simulink model "fireSpreading_analysis"  (R2021a)
settings: Solver=VariableStepAuto  StartTime=0.0  StopTime=10.0  RelTol=1e-3
values from neighbouring files (symbols this model uses):
  centroidi2 = cen_input'    [adj_cen.m]
  monitoring_critical_threshold = 15    [variables.m]
  numero_centroidi = col    [adj_cen.m]
  numero_wp = col    [adj_cen.m]
  time_burn_cell = cell_lenght*time_burn_meter    [variables.m]
  time_burn_meter = 20    [variables.m]
undefined symbols (not defined in the file or in its folder): ct, elementi_classe, pt, rt
settings Model: Creator=fiori  LastModifiedBy=fiori
settings SolverCC: AlgebraicLoopSolver=TrustRegion
settings DebuggingCC: SFMachineParentedDataDiag=warning

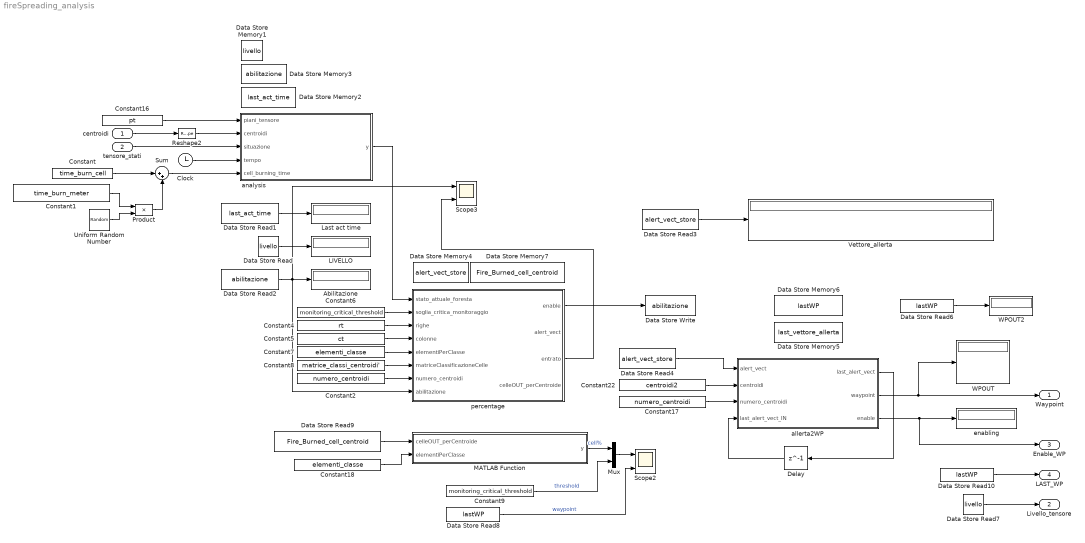
== system fireSpreading_analysis ==
  centroidi : Inport  PortDimensions=[3,numero_centroidi]
  tensore_stati : Inport  Port=2  PortDimensions=[rt,ct,pt]
  Abilitazione : Display
  Clock : Clock
  Constant : Constant  Value=time_burn_cell
  Constant1 : Constant  Value=time_burn_meter
  Constant16 : Constant  Value=pt
  Constant17 : Constant  Value=numero_centroidi
  Constant18 : Constant  Value=elementi_classe
  Constant2 : Constant  Value=numero_centroidi
  Constant22 : Constant  Value=centroidi2
  Constant4 : Constant  Value=rt
  Constant5 : Constant  Value=ct
  Constant6 : Constant  Value=monitoring_critical_threshold
  Constant7 : Constant  Value=elementi_classe
  Constant8 : Constant  Value=matrice_classi_centroidi'
  Constant9 : Constant  Value=monitoring_critical_threshold
  Data Store Memory1 : DataStoreMemory  DataStoreName=livello  ReadBeforeWriteMsg=warning  WriteAfterWriteMsg=warning  WriteAfterReadMsg=warning  ShowAdditionalParam=off  OutDataTypeStr=double
  Data Store Memory2 : DataStoreMemory  DataStoreName=last_act_time  ReadBeforeWriteMsg=warning  WriteAfterWriteMsg=warning  WriteAfterReadMsg=warning  ShowAdditionalParam=off  OutDataTypeStr=double
  Data Store Memory3 : DataStoreMemory  DataStoreName=abilitazione  ReadBeforeWriteMsg=warning  WriteAfterWriteMsg=warning  WriteAfterReadMsg=warning  ShowAdditionalParam=off  OutDataTypeStr=double
  Data Store Memory4 : DataStoreMemory  DataStoreName=alert_vect_store  ReadBeforeWriteMsg=warning  WriteAfterWriteMsg=warning  WriteAfterReadMsg=warning  ShowAdditionalParam=off  OutDataTypeStr=double  Dimensions=[1,numero_centroidi]
  Data Store Memory5 : DataStoreMemory  DataStoreName=last_vettore_allerta  ReadBeforeWriteMsg=warning  WriteAfterWriteMsg=warning  WriteAfterReadMsg=warning  ShowAdditionalParam=off  OutDataTypeStr=double  Dimensions=[1,numero_centroidi]
  Data Store Memory6 : DataStoreMemory  DataStoreName=lastWP  ReadBeforeWriteMsg=warning  WriteAfterWriteMsg=warning  WriteAfterReadMsg=warning  ShowAdditionalParam=off  OutDataTypeStr=double
  Data Store Memory7 : DataStoreMemory  DataStoreName=Fire_Burned_cell_centroid  ReadBeforeWriteMsg=warning  WriteAfterWriteMsg=warning  WriteAfterReadMsg=warning  ShowAdditionalParam=off  OutDataTypeStr=double  Dimensions=[1,numero_centroidi]
  Data Store Read : DataStoreRead  DataStoreName=livello  IndexOptions=Index vector (dialog)  Indices=1  OutputSizes=1
  Data Store Read1 : DataStoreRead  DataStoreName=last_act_time  IndexOptions=Index vector (dialog)  Indices=1  OutputSizes=1
  Data Store Read10 : DataStoreRead  DataStoreName=lastWP  IndexOptions=Index vector (dialog)  Indices=1  OutputSizes=1
  Data Store Read2 : DataStoreRead  DataStoreName=abilitazione  IndexOptions=Index vector (dialog)  Indices=1  OutputSizes=1
  Data Store Read3 : DataStoreRead  DataStoreName=alert_vect_store  IndexOptions=Index vector (dialog)  Indices=1  OutputSizes=1
  Data Store Read4 : DataStoreRead  DataStoreName=alert_vect_store  IndexOptions=Index vector (dialog)  Indices=1  OutputSizes=1
  Data Store Read6 : DataStoreRead  DataStoreName=lastWP  IndexOptions=Index vector (dialog)  Indices=1  OutputSizes=1
  Data Store Read7 : DataStoreRead  DataStoreName=livello  IndexOptions=Index vector (dialog)  Indices=1  OutputSizes=1
  Data Store Read8 : DataStoreRead  DataStoreName=lastWP  IndexOptions=Index vector (dialog)  Indices=1  OutputSizes=1
  Data Store Read9 : DataStoreRead  DataStoreName=Fire_Burned_cell_centroid  IndexOptions=Index vector (dialog)  Indices=1  OutputSizes=1
  Data Store Write : DataStoreWrite  DataStoreName=abilitazione  IndexOptions=Index vector (dialog)  Indices=1  OutputSizes=1
  Delay : Delay  DelayLength=1  InitialCondition=0
  LIVELLO : Display
  Last act time : Display
  MATLAB Function : MATLAB Function  TreatAsAtomicUnit=on
  Mux : Mux  Inputs=2
  Product : Product
  Reshape2 : Reshape  OutputDimensionality=Customize  OutputDimensions=[3,numero_wp]
  Scope2 : Scope  NumInputPorts=2
  Scope3 : Scope  NumInputPorts=3
  Sum : Sum  Inputs=|++
  Uniform Random Number : UniformRandomNumber  SampleTime=0.1
  Vettore_allerta : Display
  WPOUT : Display
  WPOUT2 : Display
  allerta2WP : MATLAB Function  TreatAsAtomicUnit=on
  analysis : MATLAB Function  TreatAsAtomicUnit=on
  enabling : Display
  percentage : MATLAB Function  TreatAsAtomicUnit=on
  Waypoint : Outport
  Livello_tensore : Outport  Port=2
  Enable_WP : Outport  Port=3
  LAST_WP : Outport  Port=4
  wires:
  centroidi/1 -> Reshape2/1
  Clock/1 -> analysis/4(tempo)
  tensore_stati/1 -> analysis/3(situazione)
  Uniform Random Number/1 -> Product/2
  Constant1/1 -> Product/1
  Constant/1 -> Sum/1
  Product/1 -> Sum/2
  analysis/1(y) -> percentage/1(stato_attuale_foresta)
  Reshape2/1 -> analysis/2(centroidi)
  Data Store Read/1 -> LIVELLO/1
  Data Store Read1/1 -> Last act time/1
  Constant6/1 -> percentage/2(soglia_critica_monitoraggio)
  Constant4/1 -> percentage/3(righe)
  Constant5/1 -> percentage/4(colonne)
  Constant7/1 -> percentage/5(elementiPerClasse)
  Constant8/1 -> percentage/6(matriceClassificazioneCelle)
  Constant2/1 -> percentage/7(numero_centroidi)
  Constant22/1 -> allerta2WP/2(centroidi)
  Data Store Read2/1 -> Scope3/1, percentage/8(abilitazione), Abilitazione/1
  percentage/1(enable) -> Data Store Write/1
  percentage/3(entrato) -> Scope3/3
  Data Store Read3/1 -> Vettore_allerta/1
  Constant16/1 -> analysis/1(piani_tensore)
  Data Store Read4/1 -> allerta2WP/1(alert_vect)
  Constant17/1 -> allerta2WP/3(numero_centroidi)
  Delay/1 -> allerta2WP/4(last_alert_vect_IN)
  allerta2WP/1(last_alert_vect) -> Delay/1
  allerta2WP/2(waypoint) -> WPOUT/1, Waypoint/1
  allerta2WP/3(enable) -> enabling/1, Enable_WP/1
  Data Store Read6/1 -> WPOUT2/1
  Data Store Read7/1 -> Livello_tensore/1
  Data Store Read9/1 -> MATLAB Function/1(celleOUT_perCentroide)
  Constant18/1 -> MATLAB Function/2(elementiPerClasse)
  Data Store Read8/1 -> Scope2/2  "waypoint"
  MATLAB Function/1(y) -> Mux/1  "cell%"
  Constant9/1 -> Mux/2  "threshold"
  Mux/1 -> Scope2/1
  Data Store Read10/1 -> LAST_WP/1
  Sum/1 -> analysis/5(cell_burning_time)

== matlab function fireSpreading_analysis/percentage ==
  settings: updateMethod=DISCRETE
  data: enable output; stato_attuale_foresta input; alert_vect output size=[1,numero_centroidi]; soglia_critica_monitoraggio input; righe input; colonne input; elementiPerClasse input; matriceClassificazioneCelle input; numero_centroidi input; abilitazione input; entrato output; celleOUT_perCentroide output size=[1,numero_centroidi]; alert_vect_store data_store_memory; Fire_Burned_cell_centroid data_store_memory
function [enable,alert_vect,entrato,celleOUT_perCentroide] = compute_Percentuale(stato_attuale_foresta,soglia_critica_monitoraggio,righe,colonne,elementiPerClasse,matriceClassificazioneCelle,numero_centroidi,abilitazione)
    global alert_vect_store;
    global Fire_Burned_cell_centroid;
    %coder.extrinsic('mat2cell');
    
    celleOUT_perCentroide=zeros(1,numero_centroidi);
    alert_vect=zeros(1,numero_centroidi);    
    
    if abilitazione==1
        for i=1:righe
            for j=1:colonne
                if stato_attuale_foresta(i,j)==3 || stato_attuale_foresta(i,j)==4
                    classe = matriceClassificazioneCelle(i,j);

                    celleOUT_perCentroide(classe) = celleOUT_perCentroide(classe) + 1;

                    if celleOUT_perCentroide(classe) >= (soglia_critica_monitoraggio * elementiPerClasse(classe))/100
                        alert_vect_store(classe)=1;
                    end
                end
            end
        end
        enable=0;
        entrato=1;
        
        Fire_Burned_cell_centroid=Fire_Burned_cell_centroid+(celleOUT_perCentroide'-Fire_Burned_cell_centroid);
    else
        enable=2;
        entrato=0;
    end
end

== matlab function fireSpreading_analysis/analysis ==
  settings: updateMethod=DISCRETE
  data: piani_tensore input; centroidi input; y output; situazione input; tempo input; livello data_store_memory; cell_burning_time input; last_act_time data_store_memory; abilitazione data_store_memory
function y = analisi_situazione(piani_tensore,centroidi,situazione,tempo,cell_burning_time)
    global livello;
    global last_act_time;
    global abilitazione;
    
    if livello==0
        livello=1;
    end
    if last_act_time==0
        last_act_time=0.1;
    end
        
    
    if ( (tempo - last_act_time) >= cell_burning_time )
        livello = livello + 1;
        if livello > piani_tensore
            livello=piani_tensore;
        end
        last_act_time = tempo;
        abilitazione = 1;
    end
    y=situazione(:,:,livello);
end

== matlab function fireSpreading_analysis/allerta2WP ==
  data: last_alert_vect output; alert_vect input size=[1,numero_centroidi]; waypoint output; centroidi input; numero_centroidi input; enable output; last_alert_vect_IN input; last_vettore_allerta data_store_memory; lastWP data_store_memory
function [last_alert_vect,waypoint,enable] = alertAnalysis(alert_vect,centroidi,numero_centroidi,last_alert_vect_IN)
    enable=0;
    waypoint=[0;0;0];
    global last_vettore_allerta;
    global lastWP;
   
    for i=1:numero_centroidi
        if alert_vect(i)==1
            if not(alert_vect(i)==last_vettore_allerta(i))
                last_vettore_allerta(i)=1;
               enable=i; 
               lastWP=i;
               break;
            else
                enable=lastWP;
            end
        end
    end
    
    
    if enable > 0 
        waypoint=centroidi(:,enable);
        enable=1;
    end
    last_alert_vect=alert_vect;
end

== matlab function fireSpreading_analysis/MATLAB Function ==
  data: celleOUT_perCentroide input; y output; elementiPerClasse input
function y = calcola_percentuale2(celleOUT_perCentroide,elementiPerClasse)
   y=(celleOUT_perCentroide*100)./elementiPerClasse; 
end
